simulink model "EL_P_test"  (R2023a)
settings: Solver=VariableStepAuto  StartTime=0.0  StopTime=0.3  RelTol=1e-3
undefined symbols (not defined in the file): Ion, Lithium
libraries: spsParallelRLCBranchLib x4, spsVoltageMeasurementLib x2, spsBatteryLib x1, spsControlledCurrentSourceLib x1, spsControlledVoltageSourceLib x1, spsCurrentMeasurementLib x1, fuzblock x1, spspowerguiLib x1
settings Model: Creator=pc180  LastModifiedBy=pc180

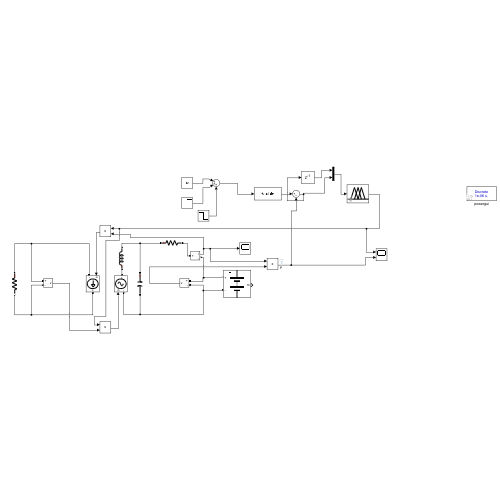
[thumbnail: Simulink's stored preview of the top-level diagram]
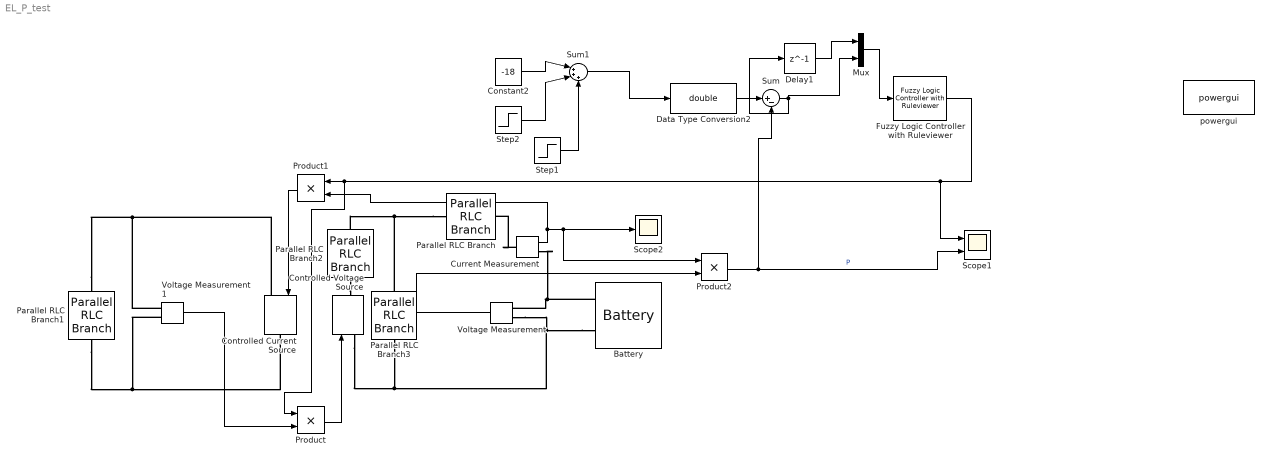
== system EL_P_test ==
  Battery : spsBatteryLib/Battery  BatType=Lithium-Ion  ShowTempParam=off  ThermalPreset=no  ShowAgeParam=off  NomV=4.2  NomQ=3.25  SOC=50  Batt_Tr=30  PresetModel=on  MaxQ=3.25  MinV=3.15  FullV=4.8887  Dis_rate=1.413  R=0.012923  Normal_OP=2.9391  expZone="[4.5376     0.15967]"  current=[6.5 13 32.5]  Units=Time  Tci=20  NomT=20  T2=-30  MaxQ2=4.8  FullV2=7.1  Normal_OP2=5.655  expZone2="[6.58           1]"  Rca=0.6  ti=2000  Dp=0  Neq0=0  Tsim=1e6  Ta1=25  Qeol=5.4*0.9  Reol=0.013333*1.2  Char_age=[2.3478, 3]  Dis_age=[2.3478, 10]  N1=1500  N2=10500  N3=1000  N4=1400  Ta2=45  N5=950
  Constant2 : Constant  Value=-18  OutDataTypeStr=single  LockScale=on
  Controlled Current Source : spsControlledCurrentSourceLib/Controlled Current Source  Initialize=on  Source_Type=AC  Amplitude=0  Phase=0  Frequency=0  Measurements=None
  Controlled Voltage Source : spsControlledVoltageSourceLib/Controlled Voltage Source  Initialize=on  Source_Type=DC  Amplitude=0  Phase=0  Frequency=0  Measurements=None
  Current Measurement : spsCurrentMeasurementLib/Current Measurement  PhasorSimulation=off  OutputType=Complex  PSBequivalent=0
  Data Type Conversion2 : DataTypeConversion  OutDataTypeStr=double  SaturateOnIntegerOverflow=off  RndMeth=Floor
  Delay1 : Delay  DelayLength=1  InitialCondition=0
  Fuzzy Logic Controller with Ruleviewer : fuzblock/Fuzzy Logic  Controller  with Ruleviewer  fismatrix=fis_power  Ts=0.0000167
  Mux : Mux  Inputs=2
  Parallel RLC Branch : spsParallelRLCBranchLib/Parallel RLC Branch  LConnTagsString=a  RConnTagsString=__new0  BranchType=R  Resistance=1  Inductance=1e-3  SetiL0=off  InitialCurrent=0  Capacitance=1e-6  Setx0=off  InitialVoltage=0  Measurements=None
  Parallel RLC Branch1 : spsParallelRLCBranchLib/Parallel RLC Branch  LConnTagsString=a  RConnTagsString=__new0  BranchType=R  Resistance=1  Inductance=1e-3  SetiL0=off  InitialCurrent=0  Capacitance=1e-6  Setx0=off  InitialVoltage=0  Measurements=None
  Parallel RLC Branch2 : spsParallelRLCBranchLib/Parallel RLC Branch  LConnTagsString=a  RConnTagsString=__new0  BranchType=L  Resistance=1  Inductance=470e-6  SetiL0=off  InitialCurrent=0  Capacitance=1e-6  Setx0=off  InitialVoltage=0  Measurements=None
  Parallel RLC Branch3 : spsParallelRLCBranchLib/Parallel RLC Branch  LConnTagsString=a  RConnTagsString=__new0  BranchType=C  Resistance=1  Inductance=1e-3  SetiL0=off  InitialCurrent=0  Capacitance=470e-6  Setx0=off  InitialVoltage=0  Measurements=None
  Product : Product
  Product1 : Product
  Product2 : Product
  Scope1 : Scope  NumInputPorts=2
  Scope2 : Scope
  Step1 : Step  Time=0.2  After=-2  SampleTime=0
  Step2 : Step  Time=0.12  After=2  SampleTime=0
  Sum : Sum  Inputs=|+-
  Sum1 : Sum  Inputs=|+++
  Voltage Measurement : spsVoltageMeasurementLib/Voltage Measurement  PhasorSimulation=off  OutputType=Complex  PSBequivalent=0
  Voltage Measurement1 : spsVoltageMeasurementLib/Voltage Measurement  PhasorSimulation=off  OutputType=Complex  PSBequivalent=0
  powergui : spspowerguiLib/powergui  Priority=1  SimulationMode=Discrete  SampleTime=1e-06  frequency=60  Iterations=50  frequencyindice=0  Pbase=100e6  ErrMax=1e-4  UnitsV=kV  UnitsW=MW  buscounter=0  FunctionMessages=off  echomessages=off  EnableUseOfTLC=off  CurrentSourceSwitches=off  DisableSnubberDevices=off  DisableRonSwitches=off  DisableVfSwitches=off  DisplayEquations=off  AutomaticDiscreteSolvers=off  SolverType=Tustin/Backward Euler (TBE)  Interpol=off  ExternalGateDelay=off  methode=off  Ts=100  x0status=blocks  SPID=on  SwTol=0  HookPort=off  NonlinearTolerance=1e-4  nMaxIteration=100  ContinueOnMaxIteration=off  RestoreLinks=warning  ResistiveCurrentMeasurement=off  Frange=[0:2:500]  Ylog=off  Xlog=on  ShowGrid=off  save=off  variable=ZData  structure=0  ZoomFFT=off  StartTime=0.0  cycles=1  DisplayStyle=1  fundamental=60  FreqAxis=off  MaxFrequency=1000  frequencyindicesteady=1  RmsSteady=1  display=off
  wires:
  Delay1/1 -> Mux/1
  Product1/1 -> Controlled Current Source/1
  Sum/1 -> Delay1/1, Mux/2
  Mux/1 -> Fuzzy Logic Controller with Ruleviewer/1
  Current Measurement/1 -> Product2/1, Scope2/1, Product1/2
  Data Type Conversion2/1 -> Sum/1
  Product2/1 -> Sum/2, Scope1/2  "P"
  Voltage Measurement1/1 -> Product/2
  Voltage Measurement/1 -> Product2/2
  Product/1 -> Controlled Voltage Source/1
  Fuzzy Logic Controller with Ruleviewer/1 -> Scope1/1, Product/1, Product1/1
  Constant2/1 -> Sum1/1
  Step1/1 -> Sum1/3
  Step2/1 -> Sum1/2
  Sum1/1 -> Data Type Conversion2/1
  connections:
  Battery/LConn2 -- Voltage Measurement/LConn2 -- Controlled Voltage Source/LConn1 -- Parallel RLC Branch3/RConn1
  Voltage Measurement/LConn1 -- Battery/LConn1 -- Current Measurement/RConn1
  Controlled Current Source/RConn1 -- Parallel RLC Branch1/RConn1 -- Voltage Measurement1/LConn2
  Parallel RLC Branch/LConn1 -- Parallel RLC Branch2/RConn1 -- Parallel RLC Branch3/LConn1
  Parallel RLC Branch1/LConn1 -- Controlled Current Source/LConn1 -- Voltage Measurement1/LConn1
  Current Measurement/LConn1 -- Parallel RLC Branch/RConn1
  Parallel RLC Branch2/LConn1 -- Controlled Voltage Source/RConn1
